simulink model "trctestJan29 1"  (R2022b)
settings: Solver=FixedStepAuto  StartTime=0.0  StopTime=inf  FixedStep=0.01  RelTol=1e-3
undefined symbols (not defined in the file): x, y, z
libraries: ros2lib x5, simulink x3, drivingvehiclecontroller x2, robotalgslib x1
settings Model: Creator=kartosis  LastModifiedBy=moham
settings OptimizationCC: EnhancedBackFolding=on  PassReuseOutputArgsAs=Individual arguments  ZeroExternalMemoryAtStartup=off  ZeroInternalMemoryAtStartup=off  MaxStackSize=64  OptimizeBlockOrder=speed  DifferentSizesBufferReuse=on  OptimizationCustomize=off  EfficientTunableParamExpr=on
settings DebuggingCC: ParameterTunabilityLossMsg=error
settings HardwareCC: ProdBitPerLong=64  ProdHWDeviceType=Intel->x86-64 (Linux 64)
settings SFSimCC: MATLABDynamicMemAlloc=off
settings RTWCC: Description=Embedded Coder  SystemTargetFile=ert.tlc  HardwareBoard=Robot Operating System 2 (ROS 2)  TLCOptions="-aInlineSetEventsForThisBaseRateFcn=TLC_FALSE -aSuppressMultiTaskScheduler=TLC_FALSE  -aRateBasedStepFcn=0"  TemplateMakefile=ert_default_tmf  Toolchain=Colcon Tools  TargetLang=C++
settings CodeAppCC: ForceParamTrailComments=on  IgnoreCustomStorageClasses=off  OperatorAnnotations=on  SimulinkDataObjDesc=on  SFDataObjDesc=on  InsertBlockDesc=on
settings ERTTargetCC: CodeInterfacePackaging=C++ class  RootIOFormat=Structure reference

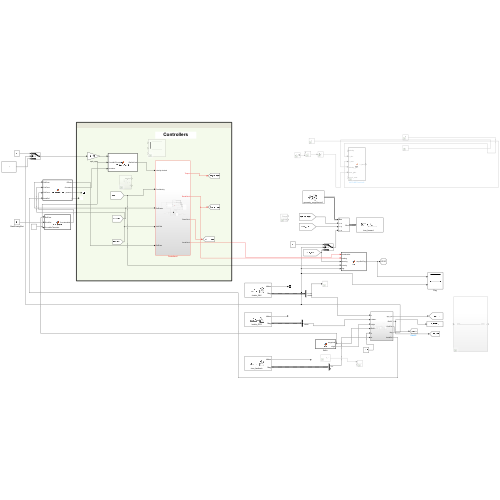
[thumbnail: Simulink's stored preview of the top-level diagram]
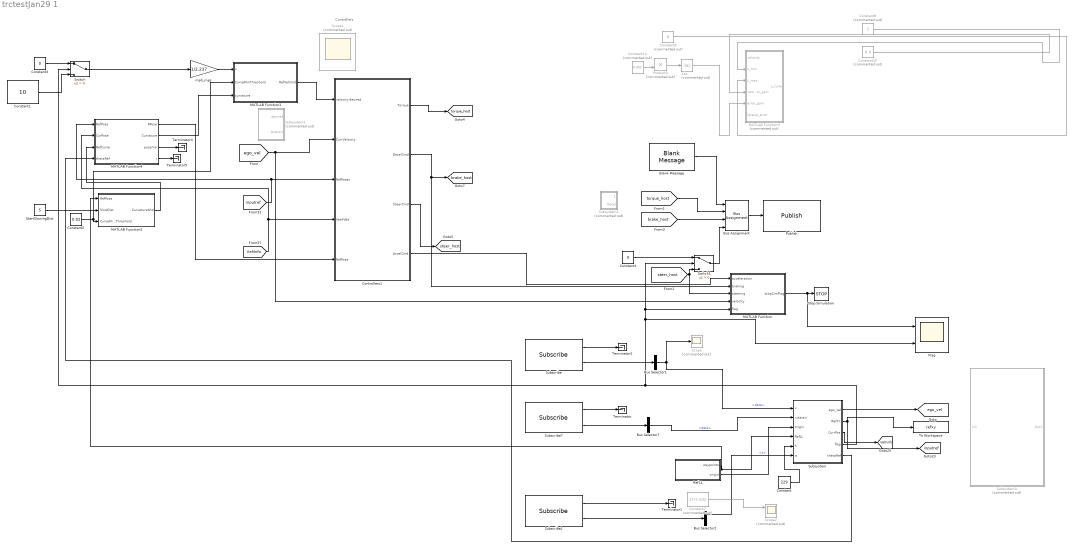
== system trctestJan29 1 ==
  note: Controllers
  Abs : Abs  Commented=on  SaturateOnIntegerOverflow=off
  Blank Message : ros2lib/Blank Message  messageClass=Message  entityType=geometry_msgs/Vector3  messageType=geometry_msgs/Vector3  SampleTime=0.01
      settings: LibrarySourceBlock=roslib/ROS 2/Blank Message
  Bus Assignment : BusAssignment  AssignedSignals=x,y,z
  Bus Selector1 : BusSelector  OutputSignals=data
  Bus Selector2 : BusSelector  OutputSignals=x,y
  Bus Selector7 : BusSelector  OutputSignals=data
  Constant : Constant  Value=229
  Constant1 : Constant  Value=10
  Constant10 : Constant  Commented=on  Value=0.4
  Constant14 : Constant  Commented=on  Value=0.032
  Constant2 : Constant  Commented=on  Value=11*1.632
  Constant3 : Constant  Value=0
  Constant4 : Constant  Value=0
  Constant5 : Constant  Value=0.02
  Constant8 : Constant  Commented=on  Value=2
  Constant9 : Constant  Commented=on  Value=6
  Controllers1 : Subsystem
  "Flag " : Scope  NumInputPorts=2
  MATLAB Function : MATLAB Function  TreatAsAtomicUnit=on
  MATLAB Function1 : MATLAB Function  TreatAsAtomicUnit=on
  MATLAB Function2 : MATLAB Function  TreatAsAtomicUnit=on
  MATLAB Function3 : MATLAB Function  Commented=on  TreatAsAtomicUnit=on
  MATLAB Function4 : MATLAB Function  TreatAsAtomicUnit=on
  Product3 : Product  Commented=on
  Publish : ros2lib/Publish  topicSource=Select from ROS network  topic=/can_forward  messageType=geometry_msgs/Vector3  QOSHistory=Keep last  QOSDepth=1  QOSReliability=Reliable  QOSDurability=Volatile
      settings: LibrarySourceBlock=roslib/ROS 2/Publish
  RefLL : MATLAB Function  TreatAsAtomicUnit=on
  Scope : Scope  Commented=on
  Scope1 : Scope  Commented=on  NumInputPorts=3
  Scope2 : Scope  Commented=on  NumInputPorts=3
  StartSlowingDist : Constant  Value=5
  Stop Simulation : Stop
  Subscribe : ros2lib/Subscribe  topicSource=Select from ROS network  topic=/matrix_IMU  messageType=std_msgs/Float64MultiArray  sampleTime=-1  QOSHistory=Keep all  QOSDepth=1  QOSReliability=Reliable  QOSDurability=Volatile
      settings: LibrarySourceBlock=roslib/ROS 2/Subscribe
  Subscribe1 : ros2lib/Subscribe  topicSource=Specify your own  topic=/can_feedback  messageType=geometry_msgs/Vector3  sampleTime=-1  QOSHistory=Keep all  QOSDepth=1  QOSReliability=Reliable  QOSDurability=Volatile
      settings: LibrarySourceBlock=roslib/ROS 2/Subscribe
  Subscribe7 : ros2lib/Subscribe  topicSource=Specify your own  topic=/matrix_GPS  messageType=std_msgs/Float64MultiArray  sampleTime=-1  QOSHistory=Keep all  QOSDepth=1  QOSReliability=Reliable  QOSDurability=Volatile
      settings: LibrarySourceBlock=roslib/ROS 2/Subscribe
  Subsystem : Subsystem
  Subsystem1 : Subsystem  Commented=on
  Subsystem2 : Subsystem  Commented=on
  Subsystem3 : Subsystem  Commented=on
  Switch : Switch  Criteria=u2 > Threshold  SaturateOnIntegerOverflow=off  InputSameDT=off
  Switch1 : Switch  Criteria=u2 > Threshold  SaturateOnIntegerOverflow=off  InputSameDT=off
  Terminator{,1..2,4..5} (5 alike) : Terminator
  To Workspace : ToWorkspace  VariableName=refxy  SaveFormat=Structure With Time  SampleTime=-1
  mph_mps : Gain  Gain=1/2.237
  tag scope: VehInfo=global, brake_host=global, ego_vel=global, inputref=global, steer_host=global, torque_host=global
  wires:
  Blank Message/1 -> Bus Assignment/1
  Bus Assignment/1 -> Publish/1
  Controllers1/1(Torque) -> [torque_host]
  [inputref] -> MATLAB Function4/1(RefPose), Controllers1/3(RefPoses)
  [VehInfo] -> MATLAB Function4/2(CurPose), Controllers1/4(VehFdbk)
  Controllers1/2(DecelCmd) -> MATLAB Function/2(braking), [brake_host]
  Controllers1/3(SteerCmd) -> [steer_host]
  Abs/1 -> MATLAB Function3/5(error_gain)
  Product3/1 -> Abs/1
  Constant10/1 -> MATLAB Function3/4(velocity_gain)
  Constant9/1 -> MATLAB Function3/3(L_max)
  Constant8/1 -> MATLAB Function3/2(L_min)
  Constant14/1 -> Product3/2
  Subscribe7/2 -> Bus Selector7/1
  Bus Selector7/1 -> Subsystem/2(<data>)  "<data>"
  RefLL/2(origin) -> Subsystem/3(origin)
  RefLL/1(waypoints) -> MATLAB Function2/1(RefPose), Subsystem/4(RefLL)
  Constant/1 -> Subsystem/5(h)
  Subsystem/1(ego_vel) -> [ego_vel]
  Subsystem/2(RefXY) -> [inputref], To Workspace/1
  Bus Selector1/1 -> Scope/1, Subsystem/1(v)  "<data>"
  Subscribe7/1 -> Terminator/1
  Subscribe/2 -> Bus Selector1/1
  Subscribe/1 -> Terminator2/1
  Subsystem/3(CurrPos) -> [VehInfo]
  [ego_vel] -> MATLAB Function/4(velocity), Controllers1/2(CurrVelocity)
  mph_mps/1 -> MATLAB Function1/1(v)
  Subscribe1/1 -> Terminator1/1
  Subscribe1/2 -> Bus Selector2/1
  [steer_host] -> Switch1/3, MATLAB Function/3(steering)
  [torque_host] -> Bus Assignment/2
  [brake_host] -> Bus Assignment/3
  Bus Selector2/1 -> Subsystem/6(w)  "<x>"
  Constant2/1 -> Scope2/1
  Subsystem/4(flag) -> "Flag "/2, MATLAB Function/5(flag), Switch1/2, Switch/2
  Constant3/1 -> Switch/1
  Constant1/1 -> Switch/3
  Switch/1 -> mph_mps/1
  Constant4/1 -> Switch1/1
  Switch1/1 -> Bus Assignment/4
  MATLAB Function/1(stopSimFlag) -> "Flag "/1, Stop Simulation/1
  Controllers1/4(AccelCmd) -> MATLAB Function/1(acceleration)
  MATLAB Function1/1(RefVelCmd) -> Controllers1/1(velocity desired)
  Constant5/1 -> MATLAB Function1/2(CurveMinThreshold), MATLAB Function2/3(CurveMinThreshold)
  StartSlowingDist/1 -> MATLAB Function2/2(SlowDist)
  MATLAB Function2/1(CurvatureAhd) -> MATLAB Function4/3(RefCurve)
  MATLAB Function4/2(Curvature) -> MATLAB Function1/3(curvature)
  MATLAB Function4/1(RPose) -> Controllers1/5(RefPose)
  MATLAB Function4/3(poserror) -> Terminator4/1
  MATLAB Function4/4(j) -> Terminator5/1
  Subsystem/5(thetaRef) -> MATLAB Function4/4(thetaRef)

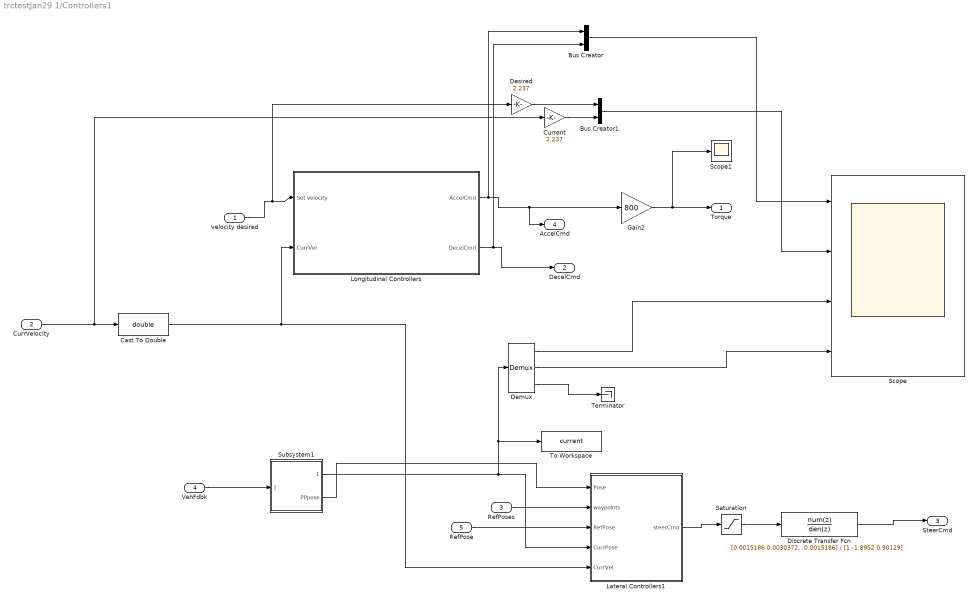
== system trctestJan29 1/Controllers1 ==
  velocity desired : Inport
  CurrVelocity : Inport  Port=2
  RefPoses : Inport  Port=3
  VehFdbk : Inport  Port=4
  RefPose : Inport  Port=5
  Bus Creator : BusCreator  Inputs=2
  Bus Creator1 : BusCreator  Inputs=2
  Cast To Double : DataTypeConversion  OutDataTypeStr=double  SaturateOnIntegerOverflow=off  RndMeth=Floor
  Current : Gain  Gain=2.237
  Demux : Demux  Outputs=3
  Desired : Gain  Gain=2.237
  Discrete Transfer Fcn : DiscreteTransferFcn  Numerator=[0.0015186 0.0030372 0.0015186]  Denominator=[1 -1.8952 0.90129]  SampleTime=0.01
  Gain2 : Gain  Gain=800
  Lateral Controllers1 : Subsystem
  Longitudinal Controllers : Subsystem
  Saturation : Saturate  UpperLimit=540  LowerLimit=-540  LinearizeAsGain=off
  Scope : Scope  NumInputPorts=4
  Scope1 : Scope
  Subsystem1 : Subsystem
  Terminator : Terminator
  To Workspace : ToWorkspace  VariableName=current  SaveFormat=Structure With Time  SampleTime=-1
  Torque : Outport
  DecelCmd : Outport  Port=2
  SteerCmd : Outport  Port=3
  AccelCmd : Outport  Port=4
  wires:
  velocity desired/1 -> Desired/1, Longitudinal Controllers/1(Set velocity)
  Longitudinal Controllers/2(DecelCmd) -> Bus Creator/2, DecelCmd/1
  Longitudinal Controllers/1(AccelCmd) -> Bus Creator/1, AccelCmd/1, Gain2/1
  CurrVelocity/1 -> Current/1, Cast To Double/1
  Subsystem1/2(PPpose) -> Lateral Controllers1/1(Pose)
  VehFdbk/1 -> Subsystem1/1(VehFdbk)
  RefPoses/1 -> Lateral Controllers1/2(waypoints)
  Cast To Double/1 -> Lateral Controllers1/5(CurrVel), Longitudinal Controllers/2(CurrVel)
  Saturation/1 -> Discrete Transfer Fcn/1
  Lateral Controllers1/1(steerCmd) -> Saturation/1
  Discrete Transfer Fcn/1 -> SteerCmd/1
  Gain2/1 -> Scope1/1, Torque/1
  Bus Creator/1 -> Scope/1
  Bus Creator1/1 -> Scope/2
  Demux/3 -> Terminator/1
  Subsystem1/1(CurrPose) -> Lateral Controllers1/4(CurrPose), Demux/1, To Workspace/1
  Demux/1 -> Scope/3
  Demux/2 -> Scope/4
  Desired/1 -> Bus Creator1/1
  Current/1 -> Bus Creator1/2
  RefPose/1 -> Lateral Controllers1/3(RefPose)

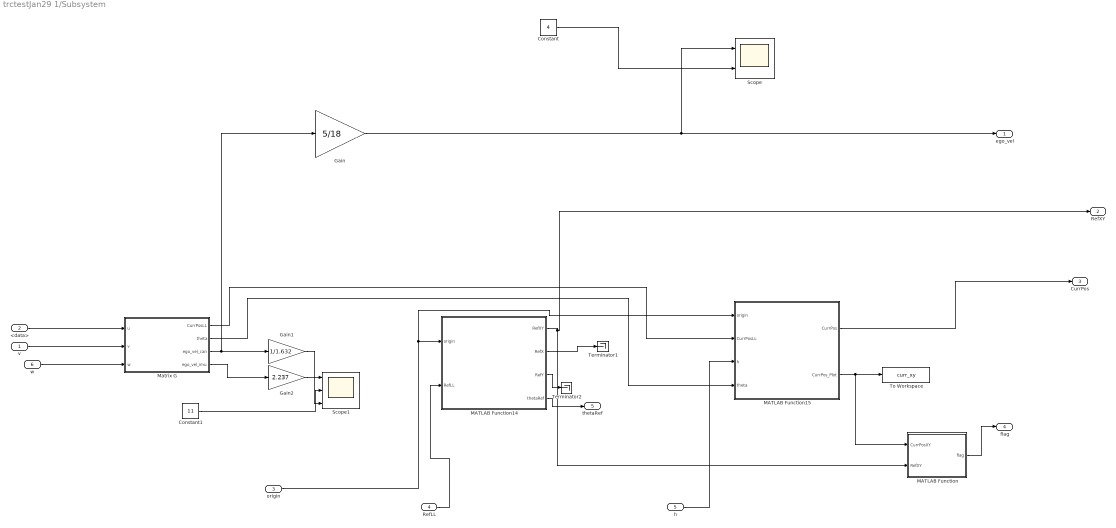
== system trctestJan29 1/Subsystem ==
  v : Inport
  <data> : Inport  Port=2
  origin : Inport  Port=3
  RefLL : Inport  Port=4
  h : Inport  Port=5
  w : Inport  Port=6
  Constant : Constant  Value=4
  Constant1 : Constant  Value=11
  Gain : Gain  Gain=5/18
  Gain1 : Gain  Gain=1/1.632
  Gain2 : Gain  Gain=2.237
  MATLAB Function : MATLAB Function  TreatAsAtomicUnit=on
  MATLAB Function14 : MATLAB Function  TreatAsAtomicUnit=on
  MATLAB Function15 : MATLAB Function  TreatAsAtomicUnit=on
  Matrix G : MATLAB Function  TreatAsAtomicUnit=on
  Scope : Scope  NumInputPorts=2
  Scope1 : Scope  NumInputPorts=3
  Terminator1 : Terminator
  Terminator2 : Terminator
  To Workspace : ToWorkspace  VariableName=curr_xy  SampleTime=-1
  ego_vel : Outport
  RefXY : Outport  Port=2
  CurrPos : Outport  Port=3
  flag : Outport  Port=4
  thetaRef : Outport  Port=5
  wires:
  <data>/1 -> Matrix G/1(u)
  MATLAB Function14/1(RefXY) -> MATLAB Function/2(RefXY), RefXY/1
  MATLAB Function14/3(RefY) -> Terminator2/1
  Matrix G/3(ego_vel_can) -> Gain/1, Gain1/1
  origin/1 -> MATLAB Function15/1(origin), MATLAB Function14/1(origin)
  Matrix G/2(theta) -> MATLAB Function15/4(theta)
  MATLAB Function15/1(CurrPos) -> CurrPos/1
  RefLL/1 -> MATLAB Function14/2(RefLL)
  h/1 -> MATLAB Function15/3(h)
  Matrix G/1(CurrPosLL) -> MATLAB Function15/2(CurrPosLL)
  MATLAB Function14/2(RefX) -> Terminator1/1
  v/1 -> Matrix G/2(v)
  Constant/1 -> Scope/2
  MATLAB Function15/2(CurrPos_Plot) -> MATLAB Function/1(CurrPosXY), To Workspace/1
  w/1 -> Matrix G/3(w)
  Matrix G/4(ego_vel_imu) -> Gain2/1
  Constant1/1 -> Scope1/2
  Gain1/1 -> Scope1/3
  Gain2/1 -> Scope1/1
  Gain/1 -> Scope/1, ego_vel/1
  MATLAB Function/1(flag) -> flag/1
  MATLAB Function14/4(thetaRef) -> thetaRef/1

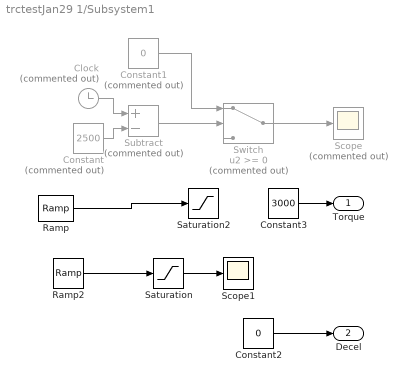
== system trctestJan29 1/Subsystem1 ==
  Clock : Clock  Commented=on
  Constant : Constant  Commented=on  Value=2500  SampleTime=0.1
  Constant1 : Constant  Commented=on  Value=0  SampleTime=0.1
  Constant2 : Constant  Value=0  SampleTime=0.01
  Constant3 : Constant  Value=3000
  Ramp : simulink/Sources/Ramp  slope=800  start=0  InitialOutput=1750
  Ramp2 : simulink/Sources/Ramp  slope=-0.05  start=2550  InitialOutput=0
  Saturation : Saturate  UpperLimit=0  LowerLimit=-5
  Saturation2 : Saturate  UpperLimit=1950  LowerLimit=0
  Scope : Scope  Commented=on
  Scope1 : Scope
  Subtract : Sum  Commented=on  Inputs=+-
  Switch : Switch  Commented=on  SaturateOnIntegerOverflow=off  InputSameDT=off
  Torque : Outport
  Decel : Outport  Port=2
  wires:
  Ramp/1 -> Saturation2/1
  Saturation/1 -> Scope1/1
  Ramp2/1 -> Saturation/1
  Clock/1 -> Subtract/1
  Constant/1 -> Subtract/2
  Subtract/1 -> Switch/2
  Switch/1 -> Scope/1
  Constant1/1 -> Switch/1
  Constant2/1 -> Decel/1
  Constant3/1 -> Torque/1

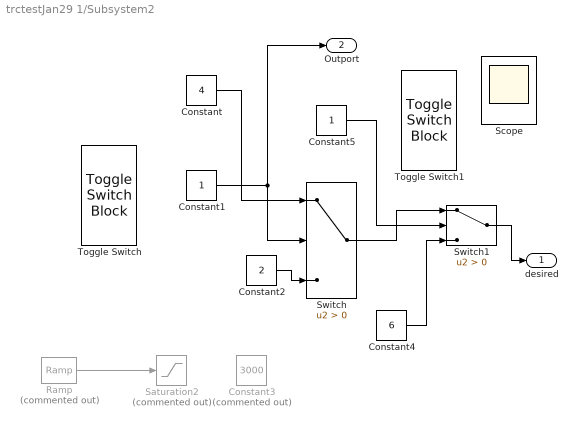
== system trctestJan29 1/Subsystem2 ==
  Constant : Constant  Value=4
  Constant1 : Constant  SampleTime=0.01
  Constant2 : Constant  Value=2
  Constant3 : Constant  Commented=on  Value=3000
  Constant4 : Constant  Value=6
  Constant5 : Constant  SampleTime=0.01
  Ramp : simulink/Sources/Ramp  Commented=on  slope=800  start=0  InitialOutput=1750
  Saturation2 : Saturate  Commented=on  UpperLimit=1950  LowerLimit=0
  Scope : Scope
  Switch : Switch  Criteria=u2 > Threshold  SaturateOnIntegerOverflow=off  InputSameDT=off
  Switch1 : Switch  Criteria=u2 > Threshold  SaturateOnIntegerOverflow=off  InputSameDT=off
  Toggle Switch : ToggleSwitchBlock
      settings: Values={{'Off', 'On'}, [0 1]}
  Toggle Switch1 : ToggleSwitchBlock
      settings: Values={{'Off', 'On'}, [0 1]}
  desired : Outport
  Outport : Outport  Port=2
  wires:
  Ramp/1 -> Saturation2/1
  Constant2/1 -> Switch/3
  Constant1/1 -> Outport/1, Switch/2
  Constant/1 -> Switch/1
  Switch1/1 -> desired/1
  Switch/1 -> Switch1/1
  Constant4/1 -> Switch1/3
  Constant5/1 -> Switch1/2

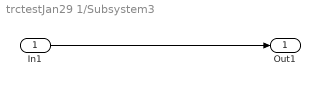
== system trctestJan29 1/Subsystem3 ==
  In1 : Inport
  Out1 : Outport
  wires:
  In1/1 -> Out1/1

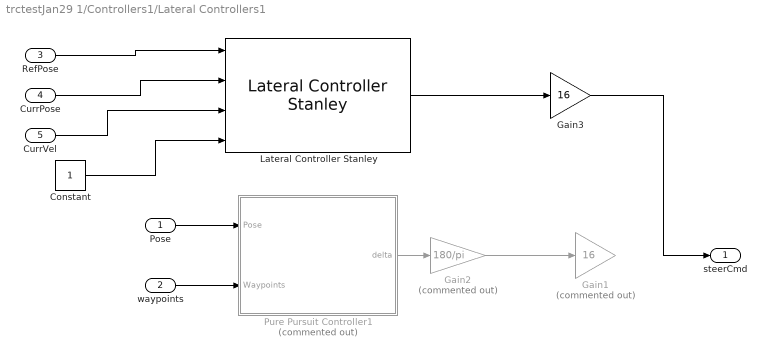
== system trctestJan29 1/Controllers1/Lateral Controllers1 ==
  Pose : Inport
  waypoints : Inport  Port=2
  RefPose : Inport  Port=3
  CurrPose : Inport  Port=4
  CurrVel : Inport  Port=5
  Constant : Constant
  Gain1 : Gain  Commented=on  Gain=16
  Gain2 : Gain  Commented=on  Gain=180/pi
  Gain3 : Gain  Gain=16
  Lateral Controller Stanley : drivingvehiclecontroller/Lateral Controller Stanley  ModelType=Kinematic bicycle model  PositionGainF=2.5  PositionGainR=2.5  YawRateGain=0.2  DelayGain=0.2  VehicleMass=1575  Lf=1.2  Lr=1.6  TireStiffness=19000  Wheelbase=2.865  MaxSteeringAngle=33
  Pure Pursuit Controller1 : Subsystem  Commented=on
  steerCmd : Outport
  wires:
  Pose/1 -> Pure Pursuit Controller1/1(Pose)
  waypoints/1 -> Pure Pursuit Controller1/2(Waypoints)
  Gain2/1 -> Gain1/1
  Pure Pursuit Controller1/1(delta) -> Gain2/1
  Lateral Controller Stanley/1 -> Gain3/1
  Gain3/1 -> steerCmd/1
  Constant/1 -> Lateral Controller Stanley/4
  RefPose/1 -> Lateral Controller Stanley/1
  CurrPose/1 -> Lateral Controller Stanley/2
  CurrVel/1 -> Lateral Controller Stanley/3

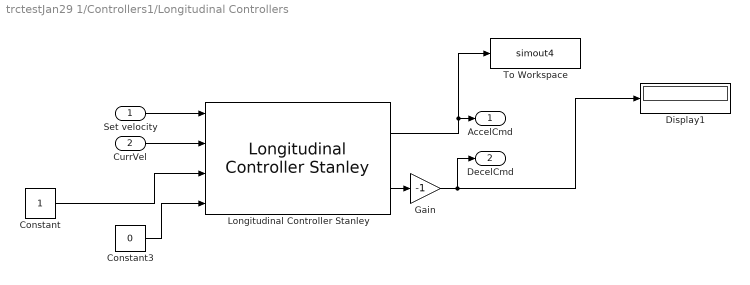
== system trctestJan29 1/Controllers1/Longitudinal Controllers ==
  Set velocity : Inport
  CurrVel : Inport  Port=2
  Constant : Constant
  Constant3 : Constant  Value=0
  Display1 : Display
  Gain : Gain  Gain=-1
  Longitudinal Controller Stanley : drivingvehiclecontroller/Longitudinal Controller Stanley  Kp=2.5  Ki=0.45  SampleTime=0.01  MaxAcceleration=2.5  MaxDeceleration=2.5
  To Workspace : ToWorkspace  VariableName=simout4  SaveFormat=Timeseries  SampleTime=-1
  AccelCmd : Outport
  DecelCmd : Outport  Port=2
  wires:
  Longitudinal Controller Stanley/2 -> Gain/1
  Gain/1 -> DecelCmd/1, Display1/1
  Longitudinal Controller Stanley/1 -> AccelCmd/1, To Workspace/1
  Set velocity/1 -> Longitudinal Controller Stanley/1
  Constant3/1 -> Longitudinal Controller Stanley/4
  Constant/1 -> Longitudinal Controller Stanley/3
  CurrVel/1 -> Longitudinal Controller Stanley/2

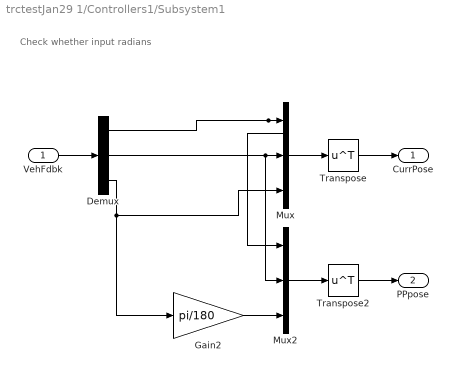
== system trctestJan29 1/Controllers1/Subsystem1 ==
  note: Check whether input radians
  VehFdbk : Inport
  Demux : Demux  Outputs=3
  Gain2 : Gain  Gain=pi/180
  Mux : Mux  Inputs=3
  Mux2 : Mux  Inputs=3
  Transpose : Math  Operator=transpose  SignedPower=on
  Transpose2 : Math  Operator=transpose  SignedPower=on
  CurrPose : Outport
  PPpose : Outport  Port=2
  wires:
  Mux/1 -> Transpose/1
  VehFdbk/1 -> Demux/1
  Demux/3 -> Mux/3, Gain2/1
  Transpose/1 -> CurrPose/1
  Mux2/1 -> Transpose2/1
  Transpose2/1 -> PPpose/1
  Demux/2 -> Mux/2, Mux2/2
  Demux/1 -> Mux2/1, Mux/1
  Gain2/1 -> Mux2/3

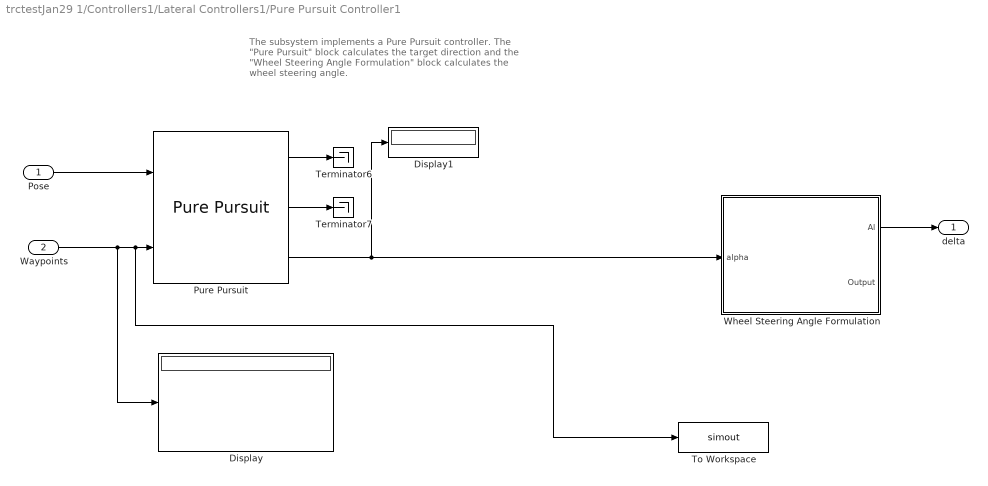
== system trctestJan29 1/Controllers1/Lateral Controllers1/Pure Pursuit Controller1 ==
  note: The subsystem implements a Pure Pursuit controller. The "Pure Pursuit" block calculates the target direction and the "Wheel Steering Angle Formulation" block calculates the wheel steering angle.
  Pose : Inport
  Waypoints : Inport  Port=2
  Display : Display
  Display1 : Display
  Pure Pursuit : robotalgslib/Pure Pursuit  DesiredLinearVelocity=5  MaxAngularVelocity=1.0  LookaheadDistance=4  TargetDirPort=on  SimulateUsing=Code generation
  Terminator6 : Terminator
  Terminator7 : Terminator
  To Workspace : ToWorkspace  VariableName=simout  SaveFormat=Timeseries  SampleTime=-1
  Wheel Steering Angle Formulation : Subsystem  mask{L=2.865, ld=4}
      mask prompts: L "Bicycle length"; ld "Lookahead distance"
      mask TypeOptions L: Bicycle length/Value
      mask TypeOptions ld: Lookahead distance/Value
      mask Display:
      | image("GeometryMask.png")
      | port_label('input', 1, 'alpha')
      | port_label('output', 1, 'delta')
  delta : Outport
  wires:
  Waypoints/1 -> To Workspace/1, Pure Pursuit/2, Display/1
  Wheel Steering Angle Formulation/1(Al) -> delta/1
  Pure Pursuit/3 -> Wheel Steering Angle Formulation/1(alpha), Display1/1
  Pure Pursuit/2 -> Terminator7/1
  Pose/1 -> Pure Pursuit/1
  Pure Pursuit/1 -> Terminator6/1

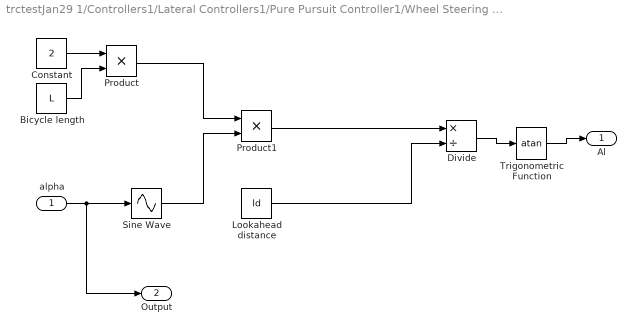
== system trctestJan29 1/Controllers1/Lateral Controllers1/Pure Pursuit Controller1/Wheel Steering Angle Formulation ==
  alpha : Inport
  Bicycle length : Constant  Value=L
  Constant : Constant  Value=2
  Divide : Product  Inputs=*/
  Lookahead distance : Constant  Value=ld
  Product : Product
  Product1 : Product
  Sine Wave : Sin  TimeSource=Use external signal  SampleTime=0
  Trigonometric Function : Trigonometry  Operator=atan
  Al : Outport
  Output : Outport  Port=2
  wires:
  Sine Wave/1 -> Product1/2
  Bicycle length/1 -> Product/2
  Constant/1 -> Product/1
  Product1/1 -> Divide/1
  Product/1 -> Product1/1
  Divide/1 -> Trigonometric Function/1
  Trigonometric Function/1 -> Al/1
  alpha/1 -> Output/1, Sine Wave/1
  Lookahead distance/1 -> Divide/2

== matlab function trctestJan29 1/Subsystem/MATLAB Function14 ==
  data: origin input; RefLL input; RefXY output; RefX output; RefY output; thetaRef output
function [RefXY,RefX,RefY, thetaRef]   = XYZenu(origin, RefLL)
%size_points = length(RefLL); %100

%zup = h*ones(size_points, 1); %100x1

%points_new = [RefLL, zup]; 

%latlong_new = points_new; 

%origin_new = latlong_new(1,:)

%origin_new = [origin(1) origin(2) origin(3)]; %1x3

xyz = lla2enu(RefLL, origin,'ellipsoid'); 
RefX = xyz(:,1);
RefY = xyz(:,2);
RefXY = [xyz(:,1) xyz(:,2)];

thetaRef = zeros(length(RefX),1); 
for i = 2:length(RefX)
    thetaRef(i,1) = atan2d((RefY(i)-RefY(i-1)),(RefX(i)-RefX(i-1)));
end
thetaRef(1) = thetaRef(2);
end

== matlab function trctestJan29 1/Subsystem/MATLAB Function15 ==
  data: CurrPos output; origin input; CurrPosLL input; h input; theta input; CurrPos_Plot output
function [CurrPos, CurrPos_Plot]  = VehicleCurrent(origin, CurrPosLL, h, theta)
zup = h; 
point_new=[CurrPosLL(1), CurrPosLL(2), zup];

x_enu = lla2enu(point_new, origin, 'ellipsoid');

head = 90 - theta;
if head < -180
   head = head + 360;
elseif abs(head) == 180
   head = abs(head);
end

CurrPos=[x_enu(1) x_enu(2) head];
CurrPos_Plot = [x_enu(1) x_enu(2)];

end

== matlab function trctestJan29 1/RefLL ==
  data: waypoints output; origin output
function [waypoints, origin] = fcn()


waypoints = [39.99787622396	-83.03295162425	229
39.99787621085	-83.03295154207	229
39.99787619776	-83.03295144561	229
39.99787618283	-83.0329513333	229
39.99787616758	-83.03295120295	229
39.99787615181	-83.0329510516	229
39.9978761336	-83.032950876	229
39.99787611409	-83.03295067282	229
39.99787609368	-83.03295043976	229
39.99787607196	-83.03295017571	229
39.99787604985	-83.03294987917	229
39.99787602683	-83.03294954927	229
39.99787600149	-83.03294918629	229
39.99787597434	-83.03294879147	229
39.99787595051	-83.03294836527	229
39.99787592815	-83.03294790727	229
39.99787590424	-83.03294741839	229
39.99787587893	-83.03294689887	229
39.99787585131	-83.03294634917	229
39.99787582058	-83.03294576861	229
39.99787578792	-83.0329451549	229
39.99787575632	-83.03294450739	229
39.99787572564	-83.03294382616	229
39.99787569452	-83.03294311202	229
39.99787566236	-83.03294236517	229
39.99787563086	-83.03294158494	229
39.9978755975	-83.03294077151	229
39.99787556024	-83.03293992438	229
39.9978755194	-83.0329390415	229
39.99787547596	-83.0329381209	229
39.99787542993	-83.03293716098	229
39.99787538388	-83.03293616139	229
39.9978753369	-83.03293512282	229
39.99787528815	-83.03293404583	229
39.99787523508	-83.03293293148	229
39.99787518049	-83.03293178189	229
39.99787512926	-83.03293059783	229
39.99787508098	-83.03292937864	229
39.99787503487	-83.03292812384	229
39.99787499096	-83.03292683235	229
39.9978749447	-83.03292550234	229
39.99787489476	-83.032924132	229
39.99787484263	-83.03292272401	229
39.99787478501	-83.03292127806	229
39.99787472268	-83.03291979518	229
39.99787465424	-83.03291827448	229
39.99787458085	-83.03291671376	229
39.99787450159	-83.032915115	229
39.99787441034	-83.03291348029	229
39.99787431791	-83.03291181653	229
39.99787424259	-83.03291013461	229
39.99787418141	-83.03290843179	229
39.99787411709	-83.03290670322	229
39.99787404932	-83.03290494552	229
39.99787399724	-83.03290315422	229
39.9978739541	-83.03290133026	229
39.99787390986	-83.03289948784	229
39.99787386648	-83.03289763135	229
39.99787382856	-83.03289574761	229
39.99787379517	-83.03289382758	229
39.99787376298	-83.03289187425	229
39.99787372443	-83.03288988986	229
39.99787367748	-83.03288787745	229
39.99787361239	-83.03288583773	229
39.99787352072	-83.03288377349	229
39.99787340786	-83.03288168517	229
39.99787329557	-83.03287956084	229
39.99787319043	-83.03287739027	229
39.99787308401	-83.03287517303	229
39.9978729819	-83.03287291005	229
39.99787289169	-83.03287061059	229
39.997872816	-83.03286827918	229
39.99787274684	-83.03286591537	229
39.99787268435	-83.03286353004	229
39.99787262376	-83.03286112507	229
39.99787256671	-83.032858697	229
39.99787250917	-83.03285625362	229
39.99787243519	-83.03285379201	229
39.9978723403	-83.03285130851	229
39.9978722358	-83.03284880261	229
39.99787213085	-83.03284627146	229
39.99787202567	-83.03284371521	229
39.99787192063	-83.03284113007	229
39.9978718137	-83.03283851652	229
39.99787171107	-83.03283587648	229
39.99787161771	-83.03283321013	229
39.99787152234	-83.03283051538	229
39.99787141746	-83.03282779672	229
39.99787131413	-83.03282505107	229
39.99787121023	-83.0328222776	229
39.99787110366	-83.03281948013	229
39.99787099056	-83.03281666482	229
39.99787087728	-83.0328138376	229
39.99787076728	-83.0328109995	229
39.99787065249	-83.03280815178	229
39.99787053336	-83.03280528834	229
39.99787042184	-83.03280240524	229
39.99787030376	-83.03279950276	229
39.99787017763	-83.03279658243	229
39.99787004689	-83.03279363904	229
39.99786991479	-83.03279067198	229
39.99786978073	-83.03278769042	229
39.99786964537	-83.03278469933	229
39.99786951026	-83.03278169967	229
39.99786938086	-83.03277869491	229
39.9978692564	-83.03277569275	229
39.99786913839	-83.03277269785	229
39.99786902032	-83.0327697103	229
39.99786889998	-83.03276672843	229
39.99786878454	-83.03276375382	229
39.99786866828	-83.03276078602	229
39.99786854073	-83.03275782349	229
39.99786840709	-83.03275486455	229
39.9978682732	-83.0327519116	229
39.99786813951	-83.03274897759	229
39.99786800589	-83.03274606362	229
39.9978678745	-83.03274315635	229
39.99786775586	-83.03274025612	229
39.99786764777	-83.03273735691	229
39.99786755125	-83.03273445782	229
39.99786746976	-83.03273155531	229
39.99786738297	-83.03272865013	229
39.99786729839	-83.03272575247	229
39.99786721173	-83.0327228756	229
39.99786710172	-83.03272000888	229
39.99786698017	-83.03271715371	229
39.99786684865	-83.03271430918	229
39.99786671158	-83.03271146411	229
39.99786657074	-83.03270861052	229
39.99786643741	-83.03270575368	229
39.99786631373	-83.03270289883	229
39.99786619637	-83.03270005351	229
39.99786608637	-83.03269721971	229
39.99786599874	-83.03269439377	229
39.99786592161	-83.03269157258	229
39.9978658257	-83.03268875565	229
39.99786570935	-83.03268593605	229
39.99786558741	-83.03268311331	229
39.9978654658	-83.03268029364	229
39.99786533812	-83.03267748634	229
39.99786520426	-83.03267468784	229
39.99786506975	-83.03267189727	229
39.99786493949	-83.03266911211	229
39.99786481546	-83.03266633535	229
39.99786469798	-83.03266356322	229
39.99786457859	-83.03266079363	229
39.99786446239	-83.03265802979	229
39.997864352	-83.03265526903	229
39.9978642417	-83.03265251072	229
39.99786412242	-83.03264975348	229
39.99786399275	-83.03264699739	229
39.99786385801	-83.03264424943	229
39.99786372142	-83.03264150975	229
39.99786358154	-83.03263877672	229
39.99786344894	-83.0326360491	229
39.99786332287	-83.03263332248	229
39.99786319822	-83.03263060152	229
39.99786307606	-83.03262788636	229
39.99786296403	-83.0326251713	229
39.99786286041	-83.03262245994	229
39.99786275472	-83.03261975736	229
39.99786263368	-83.03261706452	229
39.9978624919	-83.03261437131	229
39.99786233644	-83.03261168012	229
39.99786218076	-83.03260898941	229
39.99786203008	-83.03260629904	229
39.99786188125	-83.0326036175	229
39.99786173343	-83.03260094434	229
39.99786159629	-83.03259827475	229
39.99786147135	-83.03259561361	229
39.99786135357	-83.03259296822	229
39.99786123408	-83.03259033279	229
39.99786110781	-83.032587704	229
39.99786098065	-83.03258508032	229
39.99786084296	-83.03258245517	229
39.99786069969	-83.03257983134	229
39.99786055736	-83.03257721588	229
39.99786041603	-83.03257460837	229
39.99786027154	-83.03257200632	229
39.99786012337	-83.03256940857	229
39.99785998237	-83.03256682391	229
39.99785984183	-83.03256425381	229
39.99785970149	-83.0325616962	229
39.99785956516	-83.0325591507	229
39.99785943291	-83.03255661312	229
39.99785930467	-83.03255408342	229
39.99785917106	-83.03255156054	229
39.99785902979	-83.03254904487	229
39.99785888367	-83.03254653817	229
39.99785873796	-83.03254404238	229
39.99785858988	-83.03254155799	229
39.9978584322	-83.03253908324	229
39.99785827658	-83.03253661305	229
39.99785812695	-83.03253414314	229
39.9978579857	-83.03253168238	229
39.99785785894	-83.03252923524	229
39.99785773941	-83.03252679892	229
39.9978576203	-83.03252437419	229
39.99785750327	-83.03252195649	229
39.99785739158	-83.03251954705	229
39.99785727637	-83.03251714731	229
39.99785715496	-83.03251475355	229
39.99785703424	-83.03251236253	229
39.9978569156	-83.03250996843	229
39.99785680517	-83.03250756898	229
39.99785670259	-83.03250516328	229
39.99785660649	-83.03250275354	229
39.99785652858	-83.03250035002	229
39.99785647336	-83.03249795348	229
39.99785643972	-83.03249556488	229
39.99785642319	-83.03249317952	229
39.99785642469	-83.03249079413	229
39.99785645453	-83.03248841028	229
39.99785651276	-83.0324860248	229
39.99785659482	-83.03248362421	229
39.9978566916	-83.03248121558	229
39.99785679993	-83.03247881076	229
39.99785693051	-83.03247641523	229
39.99785708293	-83.03247402856	229
39.99785725235	-83.03247164966	229
39.9978574479	-83.0324692823	229
39.99785767473	-83.03246692458	229
39.99785792586	-83.03246456751	229
39.99785817643	-83.03246219691	229
39.99785844634	-83.03245982222	229
39.99785876575	-83.03245744159	229
39.99785913206	-83.03245506286	229
39.99785952924	-83.03245269911	229
39.99785995377	-83.03245036177	229
39.99786040527	-83.03244804451	229
39.99786088469	-83.03244574383	229
39.99786139241	-83.03244345519	229
39.9978619379	-83.03244117644	229
39.99786251991	-83.03243891439	229
39.99786312949	-83.03243667518	229
39.99786375849	-83.0324344527	229
39.99786440159	-83.03243223945	229
39.99786507112	-83.03243003987	229
39.99786578102	-83.03242786227	229
39.99786653669	-83.03242571276	229
39.99786733824	-83.03242360032	229
39.99786819312	-83.03242152589	229
39.9978690956	-83.03241948752	229
39.99787003859	-83.03241748319	229
39.99787101324	-83.03241550521	229
39.99787200961	-83.03241354986	229
39.99787303134	-83.03241161275	229
39.99787409014	-83.03240970276	229
39.99787518964	-83.03240783037	229
39.9978763296	-83.0324060054	229
39.99787749495	-83.03240421783	229
39.99787867952	-83.03240247353	229
39.99787989124	-83.03240077549	229
39.99788113368	-83.03239911581	229
39.99788240726	-83.03239749729	229
39.99788371479	-83.03239592017	229
39.99788504929	-83.03239438575	229
39.99788641527	-83.03239290016	229
39.99788780816	-83.03239146957	229
39.99788922866	-83.03239007484	229
39.99789067336	-83.03238871473	229
39.99789214572	-83.03238739831	229
39.99789364591	-83.0323861371	229
39.99789517447	-83.03238492864	229
39.99789671411	-83.03238375031	229
39.9978982593	-83.03238259835	229
39.99789981445	-83.03238148592	229
39.997901377	-83.03238041984	229
39.99790295115	-83.0323794	229
39.99790453792	-83.032378422	229
39.99790613945	-83.03237747648	229
39.99790775107	-83.03237655777	229
39.99790937817	-83.03237566418	229
39.99791101813	-83.03237479793	229
39.99791266057	-83.03237397082	229
39.99791430793	-83.03237318743	229
39.99791596055	-83.03237243626	229
39.99791761102	-83.03237170258	229
39.99791926279	-83.03237099767	229
39.99792091827	-83.03237032085	229
39.99792257474	-83.03236966002	229
39.99792423504	-83.0323690199	229
39.99792589496	-83.03236839884	229
39.9979275562	-83.03236778465	229
39.99792922134	-83.03236716812	229
39.99793088944	-83.03236654775	229
39.99793255716	-83.03236591458	229
39.99793422717	-83.03236526652	229
39.99793589359	-83.03236459361	229
39.99793755514	-83.0323639743	229
39.99793921852	-83.03236342062	229
39.99794087816	-83.03236291768	229
39.99794253741	-83.0323624602	229
39.99794420566	-83.03236204229	229
39.99794587825	-83.03236164568	229
39.99794754169	-83.03236128952	229
39.9979491983	-83.03236095525	229
39.99795085008	-83.0323606218	229
39.99795249946	-83.03236028193	229
39.99795414932	-83.03235993242	229
39.99795580101	-83.03235957698	229
39.99795745315	-83.03235922426	229
39.99795909934	-83.03235886675	229
39.99796075481	-83.03235853434	229
39.99796241548	-83.03235823777	229
39.99796407951	-83.03235797619	229
39.99796574168	-83.03235774396	229
39.99796740163	-83.03235753414	229
39.9979690586	-83.03235734742	229
39.99797071276	-83.03235718478	229
39.99797235922	-83.03235702763	229
39.99797399591	-83.03235686188	229
39.99797562007	-83.03235668328	229
39.9979772313	-83.03235648918	229
39.99797883013	-83.0323562813	229
39.9979804154	-83.03235606311	229
39.99798198761	-83.0323558369	229
39.99798355441	-83.03235560572	229
39.99798511989	-83.03235536866	229
39.99798668934	-83.03235514128	229
39.997988258	-83.03235492949	229
39.99798982816	-83.0323547296	229
39.99799139831	-83.03235454072	229
39.9979929685	-83.03235436164	229
39.99799453754	-83.03235419416	229
39.99799610239	-83.03235403149	229
39.99799765785	-83.03235386054	229
39.99799920738	-83.0323536774	229
39.99800074822	-83.03235348287	229
39.99800228273	-83.03235328702	229
39.99800381285	-83.03235308763	229
39.99800534173	-83.03235288944	229
39.99800686412	-83.03235269488	229
39.99800838236	-83.03235249807	229
39.99800990117	-83.03235228936	229
39.99801142464	-83.03235207828	229
39.99801294403	-83.03235188703	229
39.99801446512	-83.03235170398	229
39.99801598389	-83.03235151388	229
39.99801749665	-83.0323513086	229
39.99801900553	-83.03235110637	229
39.99802051334	-83.03235091399	229
39.99802201852	-83.03235072855	229
39.99802352268	-83.03235053897	229
39.99802501649	-83.03235035735	229
39.99802650069	-83.03235019019	229
39.99802797174	-83.03235001798	229
39.99802942415	-83.03234983816	229
39.99803085395	-83.03234965261	229
39.99803225783	-83.03234947437	229
39.99803363029	-83.03234929743	229
39.99803496579	-83.03234912083	229
39.99803626598	-83.03234894898	229
39.99803753096	-83.03234878666	229
39.99803875774	-83.03234862864	229
39.99803994873	-83.03234846035	229
39.99804109884	-83.03234829377	229
39.99804220739	-83.03234813766	229
39.99804327834	-83.03234799112	229
39.99804431691	-83.03234785006	229
39.998045323	-83.03234771554	229
39.99804630029	-83.03234758375	229
39.99804724531	-83.03234745279	229
39.99804815077	-83.03234732971	229
39.99804901257	-83.03234722746	229
39.99804983564	-83.03234714269	229
39.99805062048	-83.03234706641	229
39.99805137002	-83.03234699066	229
39.99805208702	-83.03234691244	229
39.99805276648	-83.03234682831	229
39.99805340126	-83.03234673647	229
39.99805399653	-83.03234663929	229
39.99805455027	-83.03234654914	229
39.99805506379	-83.03234647162	229
39.99805553948	-83.03234639864	229
39.99805597458	-83.0323463341	229
39.9980563709	-83.03234628064	229
39.9980567284	-83.03234623959	229
39.99805704719	-83.03234620473	229
39.99805732455	-83.0323461733	229
39.99805756242	-83.03234613767	229
39.99805776137	-83.03234609875	229
39.99805792138	-83.03234606248	229
39.99805804666	-83.03234602493	229
39.99805813411	-83.03234599448	229
39.99805818381	-83.03234597487	229
39.99805820051	-83.03234596212	229
39.99805818639	-83.03234595762	229
39.99805815342	-83.03234595608	229
39.99805811933	-83.03234595025	229
39.99805808764	-83.03234594499	229
39.99805806119	-83.03234593969	229
39.99805804576	-83.03234592819	229
39.99805804186	-83.03234591458	229
39.99805804767	-83.03234590354	229
39.99805805826	-83.03234589661	229
39.99805806879	-83.03234589121	229
39.99805807583	-83.03234588834	229
];
origin = waypoints(1,:);

end

== matlab function trctestJan29 1/Subsystem/MATLAB Function ==
  data: CurrPosXY input; flag output; RefXY input
function flag = fcn(CurrPosXY, RefXY)

    RefXYLast = [RefXY(end,1) RefXY(end,2)];
    
    distance = abs(sqrt((RefXYLast(1) - CurrPosXY(1)).^2 + (RefXYLast(2) - CurrPosXY(2)).^2));
    if distance < 5
        flag = 1;
    else
        flag = 0;
    end
end

== matlab function trctestJan29 1/MATLAB Function ==
  data: acceleration input; stopSimFlag output; braking input; steering input; velocity input; flag input
function stopSimFlag = fcn(acceleration, braking, steering, velocity, flag)
    
    if abs(acceleration) <= 0.01 && abs(braking) <= 0.01 && abs(steering) <= 0.01 && abs(velocity) <= 0.01 && flag == 1
        stopSimFlag = 1;
    else
        stopSimFlag = 0;
    end
end

== matlab function trctestJan29 1/MATLAB Function1 ==
  data: v input; RefVelCmd output; CurveMinThreshold input; curvature input
function RefVelCmd = VelCurveAdjust(v,CurveMinThreshold, curvature)

    if abs(curvature) >= 0 && abs(curvature) <= CurveMinThreshold
        RefVelCmd = v;
    else
        r = 1/abs(curvature);
        RefVelCmd = min(v,sqrt(9.81*r*0.9*0.4));
    end

== matlab function trctestJan29 1/MATLAB Function2 ==
  data: RefPose input; CurvatureAhd output; SlowDist input; CurveMinThreshold input
function CurvatureAhd = CurveCalc(RefPose,SlowDist,CurveMinThreshold)

DX = gradient(RefPose(:,1));
D2X = gradient(DX);
DY = gradient(RefPose(:,2));
D2Y = gradient(DY);
curvature = (DX.*D2Y - DY.*D2X) ./(DX.^2+DY.^2).^(3/2);

% calculate distance vector
distancematrix = squareform(pdist(RefPose));
distancesteps = zeros(length(RefPose)-1,1);
for i = 2:length(RefPose)
    distancesteps(i-1,1) = distancematrix(i,i-1);
end
totalDistance = sum(distancesteps); % Total distance travelled [ x y C ] 200x4
distbp = cumsum([0; distancesteps]); % Distance for each waypoint


% r = 1./abs(curvature);
% VelProfile = min(9,sqrt(9.81*r.*0.4*0.9));
st = 0;
en = 1;
j1 = 1;
CurveInfo = zeros(length(curvature),7); % [startX startY endX endY MaxCurve startidx endidx]

for j = 1:length(curvature)
    if abs(curvature(j)) >= CurveMinThreshold
        if abs(curvature(j)) >= CurveInfo(j1,5)
            CurveInfo(j1,5) = abs(curvature(j));
        end
        if st == 0
            CurveInfo(j1,1:2) = [RefPose(j,1) RefPose(j,2)]; % Startpoint
            CurveInfo(j1,6) = j;
            st = 1;
            en = 0;
        end
    elseif (abs(curvature(j)) < CurveMinThreshold) && (en == 0)
            CurveInfo(j1,3:4) = [RefPose(j,1) RefPose(j,2)]; % Endpoint
            CurveInfo(j1,7) = j;
            j1 = j1+1;
            st = 0;
            en = 1;
    end
    if (j == length(curvature)) && (en == 0)
           CurveInfo(j1,3:4) = [RefPose(j,1) RefPose(j,2)]; % Endpoint
            CurveInfo(j1,7) = j;
            j1 = j1+1;
            st = 0;
            en = 1;
    end
end
j2 = 1;
CurvatureAhd = zeros(length(curvature),1);
if j1 > 1
    for j = 1:length(distbp)
        if (distbp(j) >= (distbp(CurveInfo(j2, 6)) - SlowDist)) && (distbp(j) < distbp(CurveInfo(j2,7)))
            CurvatureAhd(j) = CurveInfo(j2,5);
        elseif (distbp(j) >= distbp(CurveInfo(j2,7))) && (j2 < j1-1)
            CurvatureAhd(j) = CurveInfo(j2,5);
            j2 = j2+1;
        else
            CurvatureAhd(j) = curvature(j);
        end
    end
end

== matlab function trctestJan29 1/MATLAB Function4 ==
  data: RefPose input; RPose output; CurPose input; RefCurve input; Curvature output; poserror output; j output; thetaRef input
function [RPose,Curvature,poserror,j] = RefPoseSearch(RefPose,CurPose, RefCurve, thetaRef)

RPose = zeros(1,3);
Curvature = 0;
m = 0; mm = 0; b = 0; bb = 0;
dist = zeros(length(RefPose),1);

for j = 1:length(RefPose)
    dist(j) = norm(CurPose(1:2) - RefPose(j,1:2));
end

[val,ind] = mink(dist,2);
j = ind(1);

if ind(1) > ind(2)
    ind = [ind(2) ;ind(1)];
end
    
m = (RefPose(ind(1),2) - RefPose(ind(2),2))/(RefPose(ind(1),1) - RefPose(ind(2),1));
if m == inf
    RPose = [RefPose(ind(1),1) CurPose(2) atan2d(RefPose(ind(2),2)-RefPose(ind(1),2),0)];
elseif m == 0
    RPose = [CurPose(1) RefPose(ind(1),2) atan2d(0,RefPose(ind(2),1)-RefPose(ind(1),1))];
else
    b = RefPose(ind(1),2) - m*RefPose(ind(1),1);
    mm = -1/m;
    bb = CurPose(2) - mm*CurPose(1);
    RPose(1:2) = [(b-bb)/(mm-m) m*((b-bb)/(mm-m))+b]; 
    RPose(3) = thetaRef(ind(1));
    Curvature = RefCurve(ind(1));

end

poserror = norm(RPose(1:2) - CurPose(1:2));

== matlab function trctestJan29 1/Subsystem/Matrix G ==
  data: u input; CurrPosLL output; theta output; ego_vel_can output; v input; w input; ego_vel_imu output
function [CurrPosLL, theta, ego_vel_can, ego_vel_imu] = fcn(u, v, w)
d = double(u(1:2));
lat = double(d(1));
long = d(2);
CurrPosLL=[lat long];

dstar = double(v(1)); %heading angle wrt north
velo = double(w(1)); %non-driven wheel speed
theta = (dstar(1)); 
ego_vel_can = double(velo(1));
ego_vel_imu = double(v(2));
end

== matlab function trctestJan29 1/MATLAB Function3 ==
  data: velocity input; L_tune output; L_min input; L_max input; velocity_gain input; error_gain input; lateral_error input
function L_tune = fcn(velocity,L_min,L_max,velocity_gain,error_gain,lateral_error)

    if velocity<=5
        L_tune = L_min;
    elseif velocity >5 && velocity<15
        L_chk = abs(velocity_gain*abs(velocity)-error_gain*lateral_error);
        if L_chk < L_min
            L_tune = L_min
        else
            L_tune = L_chk
        end
    else
        L_tune = abs(L_max-error_gain*lateral_error);
    end
